simulink model "EDR100_Model4"  (R2023a)
settings: Solver=FixedStepAuto  StartTime=0  StopTime=t_end  FixedStep=h  RelTol=1e-3
InitFcn:
  | init_Model4
values from neighbouring files (symbols this model uses):
  A_f = 2.3    [init_Model4.m]
  c_d = 0.28    [init_Model4.m]
  c_r = 9.0/1000    (= 0.009)    [init_Model4.m]
  d_wheel = 2.101/pi*0.97    (= 0.648705998746)    [init_Model4.m]
  EM_inertia = 0    [init_Model4.m]
  EM_scaling = 1.8    [init_Model4.m]
  ESS_cell_Imax = ESS_cell_Cvalue*ESS_cell_Qmax    (= 15)    [init_Model4.m]
  ESS_cell_Imin = -ESS_cell_Cvalue*ESS_cell_Qmax    (= -15)    [init_Model4.m]
  ESS_cell_Qmax = 6    [init_Model4.m]
  ESS_cell_R10 = 0.4015*ESS_cell_R_scaling/ESS_cell_Emax    (= 0.0183333333333)    [init_Model4.m]
  ESS_cell_Vmax = 4.15    [init_Model4.m]
  ESS_cell_Vmin = 2.70    (= 2.7)    [init_Model4.m]
  ESS_cells_parallel = 58    [init_Model4.m]
  ESS_cells_series = 96    [init_Model4.m]
  ESS_pack_start_voltage = interp1(ESS_cell_OCV(2,:), ESS_cell_OCV(1,:),ESS_start_SOC ) * ESS_cells_series    [init_Model4.m]
  ESS_start_SOC = 80    [init_Model4.m]
  eta_gear = 0.98    [init_Model4.m]
  g = 9.81    [init_Model4.m]
  gear_ratio = 6    [init_Model4.m]
  h = 1.0    (= 1)    [init_Model4.m]
  m_v = 1832    [init_Model4.m]
  P_aux_EM = 0    [init_Model4.m]
  P_aux_gear = 0    [init_Model4.m]
  PEC_fs = 10000    [init_Model4.m]
  PEC_i2 = PEC_i2 * PEC_scaling    [init_Model4.m]
  PEC_Imax = PEC_Imax * PEC_scaling    [init_Model4.m]
  PEC_P_aux = 0    [init_Model4.m]
  PEC_phaseCount = 3    [init_Model4.m]
  PEC_Rd_con = PEC_Rd_con / PEC_scaling    [init_Model4.m]
  PEC_Rt_con = PEC_Rt_con / PEC_scaling    [init_Model4.m]
  PEC_Tj = 100    [init_Model4.m]
  PEC_U_DC = 400    [init_Model4.m]
  PEC_Umax = PEC_U_DC    (= 400)    [init_Model4.m]
  r_wheel = d_wheel/2    (= 0.324352999373)    [init_Model4.m]
  rho = 1.225    [init_Model4.m]
  rotating_mass = 0    [init_Model4.m]
  T_EM = linspace(y0,y1,ny)    [init_Model4.m]
  T_EM_max = T_EM_raw(:,1)    [init_Model4.m]
  w_EM = linspace(x0,x1,nx)'    [init_Model4.m]
  w_EM_max = w_EM_raw(:,end)    [init_Model4.m]
  w_EM_upper = max(max(w_EM_raw))    [init_Model4.m]
undefined symbols (not defined in the file or in its folder): ESS_cell_OCV, PEC_i1, PEC_Inom, PEC_J_ON_OFF_D, PEC_J_ON_OFF_T, PEC_scaling, PEC_T1, PEC_T2, PEC_v1, PEC_Vnom
Description:
  | Simulation model 4 (fourth lecture/assignment)
  | EDR100 "Electric Drive Systems", November 2022.
  | University West, Trollhättan, Sweden
  | Developed by Stefan Skoog
settings Model: Creator=Stefan  LastModifiedBy=victo
settings OptimizationCC: ReuseModelBlockBuffer=off
settings DebuggingCC: UnconnectedInputMsg=warning  UnconnectedOutputMsg=warning  UnconnectedLineMsg=warning
settings ModelReferenceCC: EnableRefExpFcnMdlSchedulingChecks=on
settings RTWCC: DLArmComputeVersion=19.05

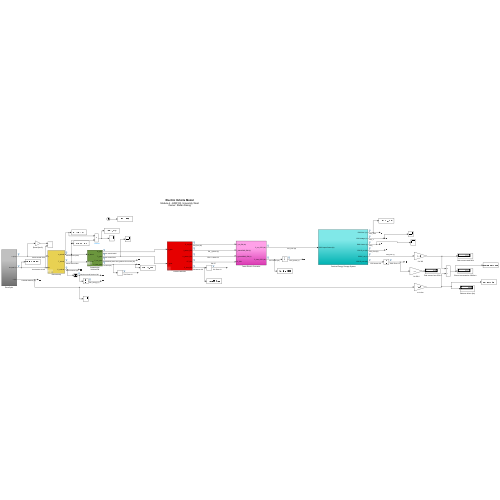
[thumbnail: Simulink's stored preview of the top-level diagram]
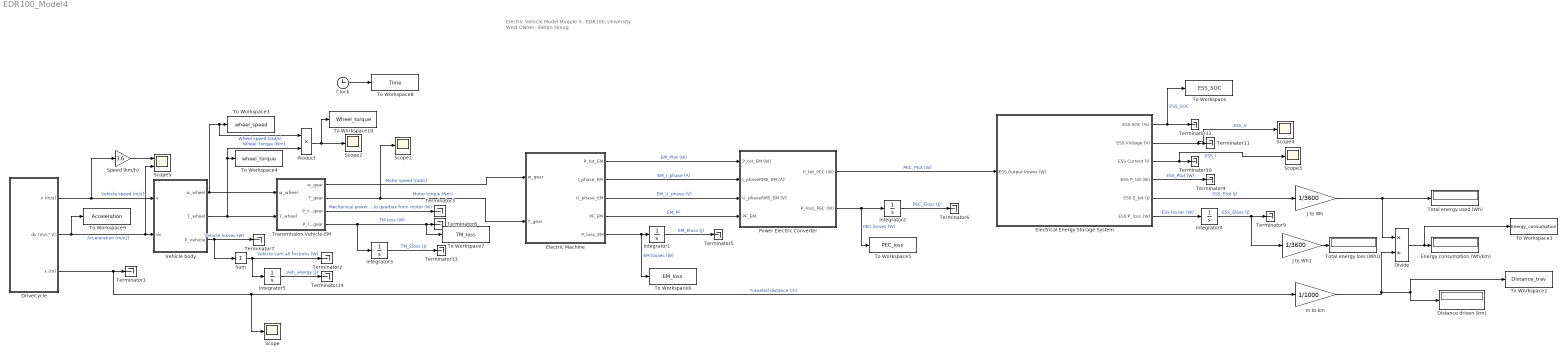
== system EDR100_Model4 ==
  note: Electric Vehicle Model
      | Module 4 - EDR100, University West
      | Owner: Stefan Skoog
  Clock : Clock
  Distance driven (km) : Display
  Divide : Product  Inputs=*/
  DriveCycle : Subsystem
  Electric Machine : Subsystem  mask{scale_EM=EM_scaling, theta_EM=EM_inertia, EM_P_aux=P_aux_EM}
      mask prompts: scale_EM "EM Scaling Factor (-)"; theta_EM "EM Inertia (kg*m²)"; EM_P_aux "Aux power (W)"
  Electrical Energy Storage System : Subsystem
  Energy consumption (Wh/km) : Display
  Integrator{1..5} (5 alike) : Integrator
  J to Wh : Gain  Gain=1/3600
  J to Wh1 : Gain  Gain=1/3600
  Power Electric Converter : Subsystem
  Product : Product  InputSameDT=on  RndMeth=Zero  SaturateOnIntegerOverflow=on  OutDataTypeStr=Inherit: Same as first input
  Scope{,1..4} (5 alike) : Scope
  Scope5 : Scope  NumInputPorts=2
  Speed (km/h) : Gain  Gain=3.6
  Sum : Sum  Inputs=+
  Terminator{1..14} (14 alike) : Terminator
  To Workspace : ToWorkspace  VariableName=ESS_SOC  SampleTime=-1
      settings: Save2DSignal=2-D array (concatenate along first dimension)
  To Workspace1 : ToWorkspace  VariableName=Energy_consumption  SampleTime=-1
      settings: Save2DSignal=2-D array (concatenate along first dimension)
  To Workspace10 : ToWorkspace  VariableName=Wheel_torque  SampleTime=-1
      settings: Save2DSignal=2-D array (concatenate along first dimension)
  To Workspace2 : ToWorkspace  VariableName=Distance_trav  SampleTime=-1
      settings: Save2DSignal=2-D array (concatenate along first dimension)
  To Workspace3 : ToWorkspace  VariableName=wheel_speed  SampleTime=-1
      settings: Save2DSignal=2-D array (concatenate along first dimension)
  To Workspace4 : ToWorkspace  VariableName=wheel_torque  SampleTime=-1
      settings: Save2DSignal=2-D array (concatenate along first dimension)
  To Workspace5 : ToWorkspace  VariableName=PEC_loss  SampleTime=-1
      settings: Save2DSignal=2-D array (concatenate along first dimension)
  To Workspace6 : ToWorkspace  VariableName=EM_loss  SampleTime=-1
      settings: Save2DSignal=2-D array (concatenate along first dimension)
  To Workspace7 : ToWorkspace  VariableName=TM_loss  SampleTime=-1
      settings: Save2DSignal=2-D array (concatenate along first dimension)
  To Workspace8 : ToWorkspace  VariableName=Time  SampleTime=-1
      settings: Save2DSignal=2-D array (concatenate along first dimension)
  To Workspace9 : ToWorkspace  VariableName=Acceleration  SampleTime=-1
      settings: Save2DSignal=2-D array (concatenate along first dimension)
  Total energy loss (Wh)1 : Display
  Total energy used (Wh) : Display
  Transmission Vehicle-EM : Subsystem  Tag=simple transmission  AncestorBlock=qss_tb_library/Gear System/Transmission  mask(Transmission){gear_ratio=gear_ratio, e_GT=eta_gear, P_GT0=P_aux_gear, w_wheel_min=1}
      mask prompts: gear_ratio "Gear ratio [-]"; e_GT "Efficiency [-]"; P_GT0 "Idling losses (friction) [W]"; w_wheel_min "Minimum wheel speed beyond which losses are generated [rad/s]"
      mask help:
      | This block simulates a transmission with a fixed gear ratio.
      |
      | Input:
      | =====
      | 	w_wheel	Speed of the wheel [rad/s]
      | 	dw_wheel	Acceleration of the wheel [rad/s^2]
      | 	T_wheel	Torque on the wheel [Nm]
      |
      | Output:
      | ======
      | 	w_trans		Speed of the fly wheel [rad/s]
      | 	dw_trans	Acceleration of the fly wheel [rad/s^2]
      | 	T_trans		Torque on the fly wheel [Nm]
  Vehicle body : Subsystem  Tag=vehicle  AncestorBlock=qss_tb_library/Vehicle/Vehicle  mask(Vehicle){m_f=m_v, mt2m_f=rotating_mass, A_f=A_f, d_wheel=d_wheel, cw=c_d, mu=c_r}
      mask prompts: m_f "Total mass of the vehicle [kg]"; mt2m_f "Rotating mass [%]"; A_f "Vehicle cross section [m^2]"; d_wheel "Wheel diameter [m]"; cw "Drag coefficient [-]"; mu "Rolling friction coefficient [-]"
      mask help:
      | This block computes the power required from the vehicle.
      |
      | Input:
      | =====
      | 	v		Speed [m/s]
      | 	dv		Acceleration [m/s^2]
      |
      | Output:
      | ======
      | 	w_wheel	Speed of the wheel [rad/s]
      | 	dw_wheel	Acceleration of the wheel [rad/s^2]
      | 	T_wheel	Torque on the wheel [Nm]
  m to km : Gain  Gain=1/1000
  wires:
  DriveCycle/2(dv (m/s^2)) -> Scope5/2, Vehicle body/2(dv), To Workspace9/1  "Acceleration (m/s2)"
  DriveCycle/1(v (m/s)) -> Vehicle body/1(v), Speed (km/h)/1  "Vehicle speed (m/s)"
  Vehicle body/1(w_wheel) -> Product/1, To Workspace3/1, Transmission Vehicle-EM/1(w_wheel)  "Wheel speed (rad/s)"
  Vehicle body/2(T_wheel) -> Product/2, To Workspace4/1, Transmission Vehicle-EM/2(T_wheel)  "Wheel Torque (Nm)"
  Vehicle body/3(P_vehicle) -> Terminator7/1, Sum/1  "Vehicle losses (W)"
  DriveCycle/3(x (m)) -> m to km/1, Scope/1, Terminator1/1  "Traveled distance (m)"
  Transmission Vehicle-EM/3(P_tot_gear) -> Terminator3/1  "Mechanical power into gearbox from motor (W)"
  Transmission Vehicle-EM/4(P_loss_gear) -> Integrator3/1, To Workspace7/1, Terminator8/1  "TM loss (W)"
  Integrator3/1 -> Terminator13/1  "TM_Eloss (J)"
  Transmission Vehicle-EM/2(T_gear) -> Scope1/1, Electric Machine/2(T_gear)  "Motor torque (Nm)"
  Integrator1/1 -> Terminator5/1  "EM_Eloss (J)"
  Electric Machine/5(P_loss_EM) -> To Workspace6/1, Integrator1/1  "EM losses (W)"
  Power Electric Converter/1(P_tot_PEC (W)) -> Electrical Energy Storage System/1(ESS Output Power (W))  "PEC_Ptot (W)"
  Electric Machine/1(P_tot_EM) -> Power Electric Converter/1(P_tot_EM (W))  "EM_Ptot (W)"
  Electric Machine/2(I_phase_EM) -> Power Electric Converter/2(I_phaseRMS_EM (A))  "EM_I_phase (A)"
  Electric Machine/3(U_phase_EM) -> Power Electric Converter/3(U_phaseRMS_EM (V))  "EM_U_phase (V)"
  Electric Machine/4(PF_EM) -> Power Electric Converter/4(PF_EM)  "EM_PF"
  Power Electric Converter/2(P_loss_PEC (W)) -> To Workspace5/1, Integrator2/1  "PEC losses (W)"
  Integrator2/1 -> Terminator6/1  "PEC_Eloss (J)"
  Integrator4/1 -> Terminator9/1, J to Wh1/1  "ESS_Eloss (J)"
  Electrical Energy Storage System/6(ESS P_loss (W)) -> Integrator4/1  "ESS losses (W)"
  Transmission Vehicle-EM/1(w_gear) -> Electric Machine/1(w_gear)  "Motor speed (rad/s)"
  m to km/1 -> Divide/2, Distance driven (km)/1, To Workspace2/1
  Electrical Energy Storage System/5(ESS E_tot (J)) -> J to Wh/1  "ESS_Etot (J)"
  J to Wh/1 -> Total energy used (Wh)/1, Divide/1
  Divide/1 -> To Workspace1/1, Energy consumption (Wh/km)/1
  Sum/1 -> Terminator2/1, Integrator5/1  "Vehicle sum all frictions (W)"
  Electrical Energy Storage System/4(ESS P_tot (W)) -> Terminator4/1  "ESS_Ptot (W)"
  Electrical Energy Storage System/2(ESS Voltage (V)) -> Scope4/1, Terminator11/1  "ESS_V"
  Electrical Energy Storage System/3(ESS Current (I)) -> Scope3/1, Terminator10/1  "ESS_I"
  Electrical Energy Storage System/1(ESS SOC (%)) -> To Workspace/1, Terminator12/1  "ESS_SOC"
  Integrator5/1 -> Terminator14/1  "Veh_energy (J)"
  Clock/1 -> To Workspace8/1
  J to Wh1/1 -> Total energy loss (Wh)1/1
  Product/1 -> To Workspace10/1, Scope2/1
  Speed (km/h)/1 -> Scope5/1

== system EDR100_Model4/DriveCycle ==
  Clock : Clock
  Differentiation : Subsystem
  Imported DriveCycle : FromWorkspace  VariableName=[t,v]  SampleTime=h  OutputAfterFinalValue=Setting to zero
  Integration : Subsystem
  To Workspace1 : ToWorkspace  VariableName=t  SampleTime=-1
  To Workspace2 : ToWorkspace  VariableName=x_tot  SampleTime=-1
  v (m/s) : Outport
  dv (m/s^2) : Outport  Port=2
  x (m) : Outport  Port=3  InitialOutput=0
  wires:
  Clock/1 -> To Workspace1/1  "Time (s)"
  Imported DriveCycle/1 -> Differentiation/1(V_z), Integration/1(V_z), v (m/s)/1  "Speed (m/s)"
  Integration/1(x_tot1) -> To Workspace2/1, x (m)/1  "Distance (m)"
  Differentiation/1(D_z) -> dv (m/s^2)/1  "Acceleration (m/s2)"

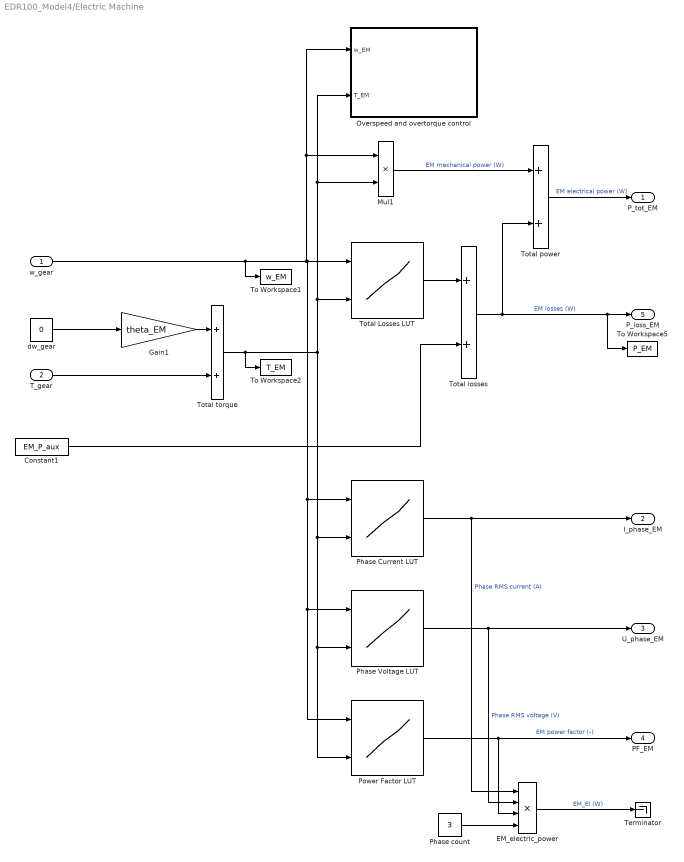
== system EDR100_Model4/Electric Machine ==
  w_gear : Inport
  T_gear : Inport  Port=2
  Constant1 : Constant  Value=EM_P_aux
  EM_electric_power : Product  Inputs=4
  Gain1 : Gain  Gain=theta_EM  SaturateOnIntegerOverflow=on  OutDataTypeStr=Inherit: Same as input  ParamDataTypeStr=Inherit: Same as input
  Mul1 : Product  Inputs=**
  Overspeed and overtorque control : Subsystem
  Phase Current LUT : Lookup_n-D  BreakpointsForDimension1=w_EM  BreakpointsForDimension2=T_EM  Table=Iph_EM_map'  ExtrapMethod=Clip  InternalRulePriority=Speed  RndMeth=Simplest
      settings: InputPortMap=u0,u1
  Phase Voltage LUT : Lookup_n-D  BreakpointsForDimension1=w_EM  BreakpointsForDimension2=T_EM  Table=Uph_EM_map'  ExtrapMethod=Clip  InternalRulePriority=Speed  RndMeth=Simplest
      settings: InputPortMap=u0,u1
  Phase count : Constant  Value=3
  Power Factor LUT : Lookup_n-D  BreakpointsForDimension1=w_EM  BreakpointsForDimension2=T_EM  Table=PF_EM_map'  ExtrapMethod=Clip  InternalRulePriority=Speed  RndMeth=Simplest
      settings: InputPortMap=u0,u1
  Terminator : Terminator
  To Workspace1 : ToWorkspace  VariableName=w_EM  SampleTime=-1
  To Workspace2 : ToWorkspace  VariableName=T_EM  SampleTime=-1
  To Workspace5 : ToWorkspace  VariableName=P_EM  SampleTime=-1
  Total Losses LUT : Lookup_n-D  BreakpointsForDimension1=w_EM  BreakpointsForDimension2=T_EM  Table=Loss_EM_map'  ExtrapMethod=Clip  InternalRulePriority=Speed  RndMeth=Simplest
      settings: InputPortMap=u0,u1
  Total losses : Sum  InputSameDT=on  SaturateOnIntegerOverflow=on  OutDataTypeStr=Inherit: Same as first input
  Total power : Sum  InputSameDT=on  SaturateOnIntegerOverflow=on  OutDataTypeStr=Inherit: Same as first input
  Total torque : Sum  InputSameDT=on  SaturateOnIntegerOverflow=on  OutDataTypeStr=Inherit: Same as first input
  dw_gear : Constant  Value=0
  P_tot_EM : Outport
  I_phase_EM : Outport  Port=2
  U_phase_EM : Outport  Port=3
  PF_EM : Outport  Port=4
  P_loss_EM : Outport  Port=5
  wires:
  T_gear/1 -> Total torque/2
  dw_gear/1 -> Gain1/1
  w_gear/1 -> To Workspace1/1, Total Losses LUT/1, Phase Current LUT/1, Power Factor LUT/1, Phase Voltage LUT/1, Overspeed and overtorque control/1(w_EM), Mul1/1
  Total losses/1 -> Total power/2, P_loss_EM/1, To Workspace5/1  "EM losses (W)"
  Total Losses LUT/1 -> Total losses/1
  Gain1/1 -> Total torque/1
  Total torque/1 -> Phase Current LUT/2, Power Factor LUT/2, Phase Voltage LUT/2, Total Losses LUT/2, Overspeed and overtorque control/2(T_EM), Mul1/2, To Workspace2/1
  Constant1/1 -> Total losses/2
  Phase Current LUT/1 -> I_phase_EM/1, EM_electric_power/1  "Phase RMS current (A)"
  Phase Voltage LUT/1 -> U_phase_EM/1, EM_electric_power/2  "Phase RMS voltage (V)"
  Total power/1 -> P_tot_EM/1  "EM electrical power (W)"
  Mul1/1 -> Total power/1  "EM mechanical power (W)"
  Power Factor LUT/1 -> PF_EM/1, EM_electric_power/3  "EM power factor (-)"
  EM_electric_power/1 -> Terminator/1  "EM_El (W)"
  Phase count/1 -> EM_electric_power/4

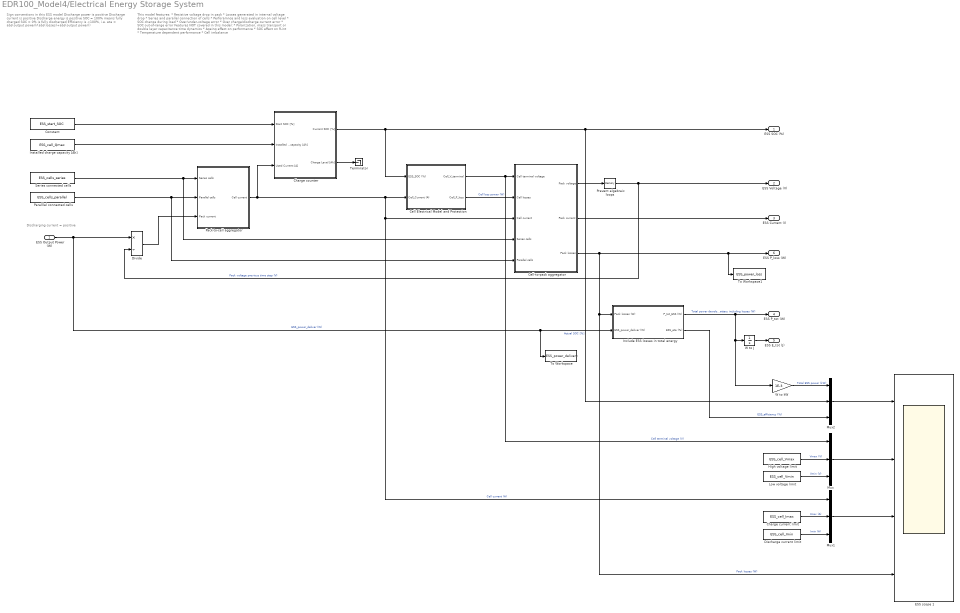
== system EDR100_Model4/Electrical Energy Storage System ==
  note: Discharging current = positive
  note: This model features:
      | * Resistive voltage drop in pack
      | * Losses generated in internal voltage drop
      | * Series and parallel connection of cells
      | * Perforamnce and loss evaluation on cell level
      | * SOC change during load
      | * Over/under-voltage error
      | * Over charge/discharge current error
      | * SOC out-of-range error
      |
      | Features NOT covered in this model:
      | * Polarization, mass transport or double layer capacitance time dynamics
      | * Ageing effect on performance
      | * SOC effect on R-int
      | * Temperature dependent performance
      | * Cell imbalance
  note: Sign conventions in this ESS model
      | Discharge power is positive
      | Discharge current is positive
      | Discharge energy is positive
      | SOC = 100% means fully charged
      | SOC = 0% is fully discharged
      | Efficiency is <100%, i.e.
      | eta = abs(output power)/(abs(losses)+abs(output power))
  ESS Output Power (W) : Inport
  Cell Electrical Model and Protection : Subsystem
  Cell-to-pack aggregator : Subsystem
  Charge counter : Subsystem
  Charge current limit : Constant  Value=ESS_cell_Imax
  Constant : Constant  Value=ESS_start_SOC
  Discharge current limit : Constant  Value=ESS_cell_Imin
  Divide : Product  Inputs=*/
  ESS scope 1 : Scope  NumInputPorts=4
  High voltage limit : Constant  Value=ESS_cell_Vmax
  Include ESS losses in total energy : Subsystem
  Installed charge capacity [Ah] : Constant  Value=ESS_cell_Qmax
  Low voltage limit : Constant  Value=ESS_cell_Vmin
  Mux : Mux  Inputs=3
  Mux1 : Mux  Inputs=3
  Mux2 : Mux  Inputs=3
  Pack-to-cell aggregator : Subsystem
  Paralllel connected cells : Constant  Value=ESS_cells_parallel
  Prevent algebraic loops : Memory  InitialCondition=ESS_pack_start_voltage
  Series connected cells : Constant  Value=ESS_cells_series
  Terminator : Terminator
  To Workspace : ToWorkspace  VariableName=ESS_power_delivery  SampleTime=-1
      settings: Save2DSignal=2-D array (concatenate along first dimension)
  To Workspace1 : ToWorkspace  VariableName=ESS_power_loss  SampleTime=-1
      settings: Save2DSignal=2-D array (concatenate along first dimension)
  W to J : Integrator
  W to kW : Gain  Gain=1E-3
  ESS SOC (%) : Outport
  ESS Voltage (V) : Outport  Port=2
  ESS Current (I) : Outport  Port=3
  ESS P_tot (W) : Outport  Port=4
  ESS E_tot (J) : Outport  Port=5
  ESS P_loss (W) : Outport  Port=6
  wires:
  Series connected cells/1 -> Cell-to-pack aggregator/4(Series cells), Pack-to-cell aggregator/1(Series cells)
  Pack-to-cell aggregator/1(Cell current) -> Mux1/1, Cell-to-pack aggregator/3(Cell current), Cell Electrical Model and Protection/2(Cell_Current (A)), Charge counter/3(Used Current [A])  "Cell current (A)"
  Installed charge capacity [Ah]/1 -> Charge counter/2(Installed charge capacity [Ah])
  Constant/1 -> Charge counter/1(Start SOC [%])
  Divide/1 -> Pack-to-cell aggregator/3(Pack current)
  Paralllel connected cells/1 -> Cell-to-pack aggregator/5(Parallel cells), Pack-to-cell aggregator/2(Parallel cells)
  Charge counter/1(Current SOC [%]) -> ESS SOC (%)/1, Mux2/2, Cell Electrical Model and Protection/1(ESS_SOC (%))  "Actual SOC [%]"
  Charge counter/2(Charge Level [Ah]) -> Terminator/1
  Cell Electrical Model and Protection/1(Cell_V_terminal) -> Mux/1, Cell-to-pack aggregator/1(Cell terminal voltage)  "Cell terminal voltage (V)"
  Cell Electrical Model and Protection/2(Cell_P_loss) -> Cell-to-pack aggregator/2(Cell losses)  "Cell loss power (W)"
  Cell-to-pack aggregator/3(Pack losses) -> To Workspace1/1, ESS P_loss (W)/1, Include ESS losses in total energy/1(Pack losses (W)), ESS scope 1/4  "Pack losses (W)"
  Cell-to-pack aggregator/1(Pack voltage) -> Prevent algebraic loops/1
  Prevent algebraic loops/1 -> ESS Voltage (V)/1, Divide/2  "Pack voltage previous time step (V)"
  Cell-to-pack aggregator/2(Pack current) -> ESS Current (I)/1
  ESS Output Power (W)/1 -> Divide/1, To Workspace/1, Include ESS losses in total energy/2(ESS_power_deliver (W))  "ESS_power_deliver (W)"
  Mux2/1 -> ESS scope 1/1
  Mux/1 -> ESS scope 1/2
  Mux1/1 -> ESS scope 1/3
  W to J/1 -> ESS E_tot (J)/1
  Include ESS losses in total energy/1(P_tot_ESS (W)) -> ESS P_tot (W)/1, W to kW/1, W to J/1  "Total power developed in battery including losses (W)"
  Charge current limit/1 -> Mux1/2  "Imax (A)"
  High voltage limit/1 -> Mux/2  "Vmax (V)"
  Discharge current limit/1 -> Mux1/3  "Imin (A)"
  Low voltage limit/1 -> Mux/3  "Vmin (V)"
  Include ESS losses in total energy/2(ESS_eta (%)) -> Mux2/3  "ESS_efficiency (%)"
  W to kW/1 -> Mux2/1  "Total ESS power (kW)"

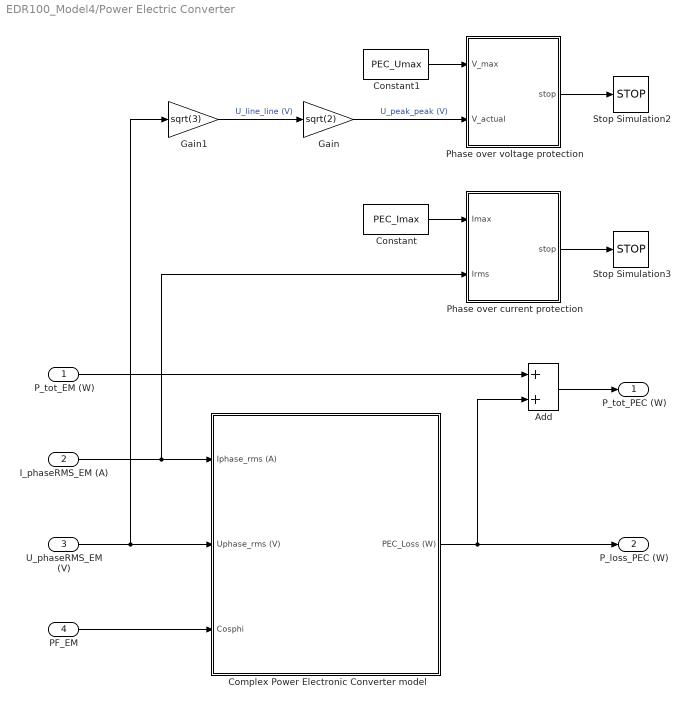
== system EDR100_Model4/Power Electric Converter ==
  P_tot_EM (W) : Inport
  I_phaseRMS_EM (A) : Inport  Port=2
  U_phaseRMS_EM (V) : Inport  Port=3
  PF_EM : Inport  Port=4
  Add : Sum
  Complex Power Electronic Converter model : Subsystem  mask(3-phase IGBT inverter){scale_PEC=PEC_scaling, Udc=PEC_U_DC, fsw=PEC_fs, Tjunct=PEC_Tj, LV_Losses=PEC_P_aux}
      mask prompts: scale_PEC "PEC Scaling Factor (-)"; Udc "Supply direct voltage level (V)"; fsw "Switching frequency (Hz)"; Tjunct "IGBT Junction temperature (°C)"; LV_Losses "Aux losses (W)"
      mask help:
      | This blocks simulates losses for a three-leg, two-level converter based on forward conduction losses and diod losses in IGBT modules.
      |
      | Input:
      | =====
      | I_phaseRMS		Phase RMS current of electric machine (V)
      | U_phaseRMS		Phase RMS voltage of electric machine (V)
      | cosphi			Power factor [0..1] of electric machine (-)
      |
      | Ouput:
      | ======
      | Pinv	Total losses in inverter (W)
  Constant : Constant  Value=PEC_Imax
  Constant1 : Constant  Value=PEC_Umax
  Gain : Gain  Gain=sqrt(2)
  Gain1 : Gain  Gain=sqrt(3)
  Phase over current protection : MATLAB Function  TreatAsAtomicUnit=on
  Phase over voltage protection : MATLAB Function  TreatAsAtomicUnit=on
  Stop Simulation2 : Stop
  Stop Simulation3 : Stop
  P_tot_PEC (W) : Outport
  P_loss_PEC (W) : Outport  Port=2
  wires:
  Constant/1 -> Phase over current protection/1(Imax)
  Constant1/1 -> Phase over voltage protection/1(V_max)
  PF_EM/1 -> Complex Power Electronic Converter model/3(Cosphi)
  P_tot_EM (W)/1 -> Add/1
  Phase over current protection/1(stop) -> Stop Simulation3/1
  Add/1 -> P_tot_PEC (W)/1
  Gain1/1 -> Gain/1  "U_line_line (V)"
  Phase over voltage protection/1(stop) -> Stop Simulation2/1
  Gain/1 -> Phase over voltage protection/2(V_actual)  "U_peak_peak (V)"
  U_phaseRMS_EM (V)/1 -> Gain1/1, Complex Power Electronic Converter model/2(Uphase_rms (V))
  I_phaseRMS_EM (A)/1 -> Phase over current protection/2(Irms), Complex Power Electronic Converter model/1(Iphase_rms (A))
  Complex Power Electronic Converter model/1(PEC_Loss (W)) -> Add/2, P_loss_PEC (W)/1

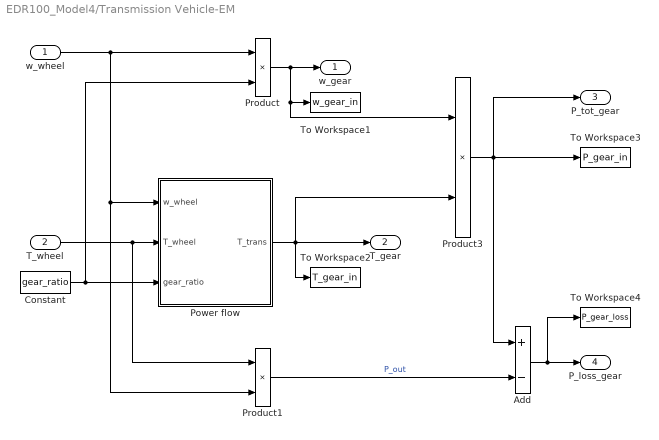
== system EDR100_Model4/Transmission Vehicle-EM ==
  w_wheel : Inport
  T_wheel : Inport  Port=2
  Add : Sum  Inputs=+-
  Constant : Constant  Value=gear_ratio
  Power flow : Subsystem
  Product : Product  InputSameDT=on  RndMeth=Zero  SaturateOnIntegerOverflow=on  OutDataTypeStr=Inherit: Same as first input
  Product1 : Product  InputSameDT=on  RndMeth=Zero  SaturateOnIntegerOverflow=on  OutDataTypeStr=Inherit: Same as first input
  Product3 : Product  InputSameDT=on  RndMeth=Zero  SaturateOnIntegerOverflow=on  OutDataTypeStr=Inherit: Same as first input
  To Workspace1 : ToWorkspace  VariableName=w_gear_in  SampleTime=-1
  To Workspace2 : ToWorkspace  VariableName=T_gear_in  SampleTime=-1
  To Workspace3 : ToWorkspace  VariableName=P_gear_in  SampleTime=-1
  To Workspace4 : ToWorkspace  VariableName=P_gear_loss  SampleTime=-1
  w_gear : Outport  InitialOutput=0
  T_gear : Outport  Port=2  InitialOutput=0
  P_tot_gear : Outport  Port=3  InitialOutput=0
  P_loss_gear : Outport  Port=4  InitialOutput=0
  wires:
  Product3/1 -> P_tot_gear/1, To Workspace3/1, Add/1
  w_wheel/1 -> Product1/2, Power flow/1(w_wheel), Product/1
  Constant/1 -> Product/2, Power flow/3(gear_ratio)
  T_wheel/1 -> Product1/1, Power flow/2(T_wheel)
  Product/1 -> Product3/1, To Workspace1/1, w_gear/1
  Power flow/1(T_trans) -> Product3/2, To Workspace2/1, T_gear/1
  Product1/1 -> Add/2  "P_out"
  Add/1 -> To Workspace4/1, P_loss_gear/1

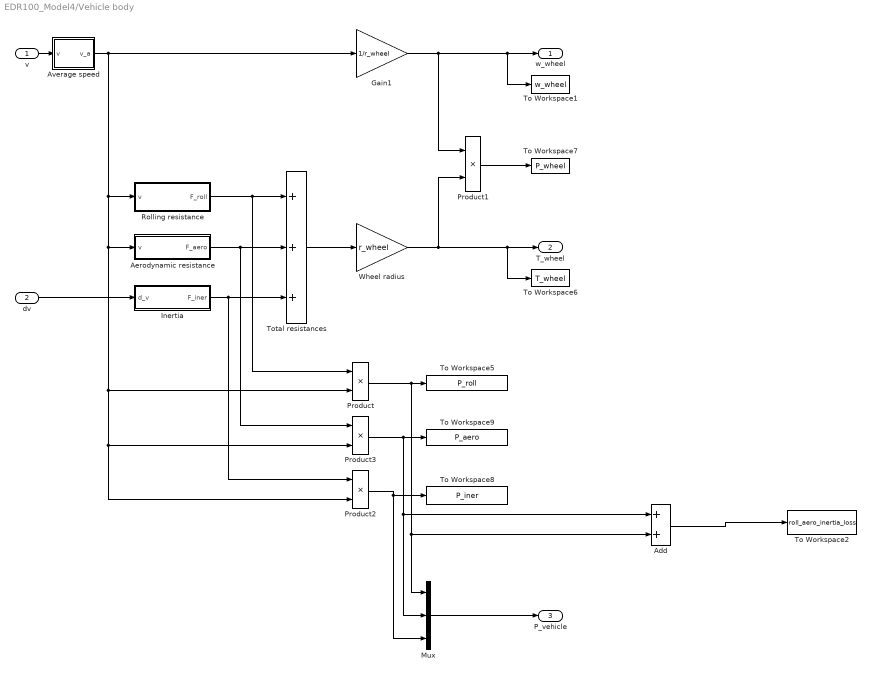
== system EDR100_Model4/Vehicle body ==
  v : Inport
  dv : Inport  Port=2
  Add : Sum
  Aerodynamic resistance : Subsystem
  Average speed : Subsystem
  Gain1 : Gain  Gain=1/r_wheel  SaturateOnIntegerOverflow=on  OutDataTypeStr=Inherit: Same as input  ParamDataTypeStr=Inherit: Same as input
  Inertia : Subsystem
  Mux : Mux  Inputs=3
  Product{,1..3} (4 alike) : Product  InputSameDT=on  RndMeth=Zero  SaturateOnIntegerOverflow=on  OutDataTypeStr=Inherit: Same as first input
  Rolling resistance : Subsystem
  To Workspace1 : ToWorkspace  VariableName=w_wheel  SampleTime=-1
  To Workspace2 : ToWorkspace  VariableName=roll_aero_inertia_loss  SampleTime=-1
      settings: Save2DSignal=2-D array (concatenate along first dimension)
  To Workspace5 : ToWorkspace  VariableName=P_roll  SampleTime=-1
  To Workspace6 : ToWorkspace  VariableName=T_wheel  SampleTime=-1
  To Workspace7 : ToWorkspace  VariableName=P_wheel  SampleTime=-1
  To Workspace8 : ToWorkspace  VariableName=P_iner  SampleTime=-1
  To Workspace9 : ToWorkspace  VariableName=P_aero  SampleTime=-1
  Total resistances : Sum  Inputs=+++  InputSameDT=on  SaturateOnIntegerOverflow=on  OutDataTypeStr=Inherit: Same as first input
  Wheel radius : Gain  Gain=r_wheel  SaturateOnIntegerOverflow=on  OutDataTypeStr=Inherit: Same as input  ParamDataTypeStr=Inherit: Same as input
  w_wheel : Outport  InitialOutput=0
  T_wheel : Outport  Port=2  InitialOutput=0
  P_vehicle : Outport  Port=3  InitialOutput=0
  wires:
  Product/1 -> To Workspace5/1, Add/2, Mux/1
  Product1/1 -> To Workspace7/1
  Product3/1 -> Mux/2, Add/1, To Workspace9/1
  Product2/1 -> Mux/3, To Workspace8/1
  v/1 -> Average speed/1(v)
  dv/1 -> Inertia/1(d_v)
  Wheel radius/1 -> Product1/2, To Workspace6/1, T_wheel/1
  Total resistances/1 -> Wheel radius/1
  Inertia/1(F_iner) -> Product2/1, Total resistances/3
  Aerodynamic resistance/1(F_aero) -> Total resistances/2, Product3/1
  Rolling resistance/1(F_roll) -> Product/1, Total resistances/1
  Gain1/1 -> To Workspace1/1, w_wheel/1, Product1/1
  Average speed/1(v_a) -> Product/2, Product2/2, Product3/2, Aerodynamic resistance/1(v), Rolling resistance/1(v), Gain1/1
  Mux/1 -> P_vehicle/1
  Add/1 -> To Workspace2/1

== system EDR100_Model4/DriveCycle/Differentiation ==
  V_z : Inport
  Sum1 : Sum  Inputs=+-  InputSameDT=on  SaturateOnIntegerOverflow=on  OutDataTypeStr=Inherit: Same as first input
  Unit Delay1 : UnitDelay  SampleTime=h
  D_z : Outport  InitialOutput=0
  wires:
  Unit Delay1/1 -> Sum1/2
  V_z/1 -> Sum1/1, Unit Delay1/1
  Sum1/1 -> D_z/1

== system EDR100_Model4/DriveCycle/Integration ==
  V_z : Inport
  Gain4 : Gain  Gain=0.5*h  SaturateOnIntegerOverflow=on  OutDataTypeStr=Inherit: Same as input  ParamDataTypeStr=Inherit: Same as input
  Plant : UnitDelay  InitialCondition=1  SampleTime=h
  Sum2 : Sum  InputSameDT=on  SaturateOnIntegerOverflow=on  OutDataTypeStr=Inherit: Same as first input
  Sum4 : Sum  InputSameDT=on  SaturateOnIntegerOverflow=on  OutDataTypeStr=Inherit: Same as first input
  Unit Delay2 : UnitDelay  SampleTime=h
  x_tot1 : Outport  InitialOutput=0
  wires:
  Unit Delay2/1 -> Sum2/2
  Sum2/1 -> Gain4/1
  Gain4/1 -> Sum4/2
  Plant/1 -> x_tot1/1, Sum4/1
  V_z/1 -> Sum2/1, Unit Delay2/1
  Sum4/1 -> Plant/1

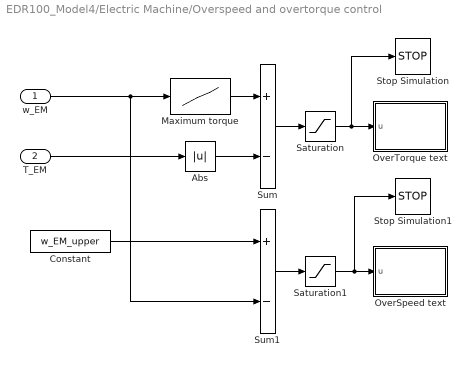
== system EDR100_Model4/Electric Machine/Overspeed and overtorque control ==
  w_EM : Inport
  T_EM : Inport  Port=2
  Abs : Abs
  Constant : Constant  Value=w_EM_upper
  Maximum torque : Lookup  InputValues=w_EM_max  Table=T_EM_max
  OverSpeed text : MATLAB Function  TreatAsAtomicUnit=on
  OverTorque text : MATLAB Function  TreatAsAtomicUnit=on
  Saturation : Saturate  UpperLimit=0  LowerLimit=-inf
  Saturation1 : Saturate  UpperLimit=0  LowerLimit=-inf
  Stop Simulation : Stop
  Stop Simulation1 : Stop
  Sum : Sum  Inputs=+-  InputSameDT=on  SaturateOnIntegerOverflow=on  OutDataTypeStr=Inherit: Same as first input
  Sum1 : Sum  Inputs=+-  InputSameDT=on  SaturateOnIntegerOverflow=on  OutDataTypeStr=Inherit: Same as first input
  wires:
  Saturation/1 -> Stop Simulation/1, OverTorque text/1(u)
  Constant/1 -> Sum1/1
  w_EM/1 -> Maximum torque/1, Sum1/2
  Abs/1 -> Sum/2
  Saturation1/1 -> Stop Simulation1/1, OverSpeed text/1(u)
  Sum1/1 -> Saturation1/1
  T_EM/1 -> Abs/1
  Maximum torque/1 -> Sum/1
  Sum/1 -> Saturation/1

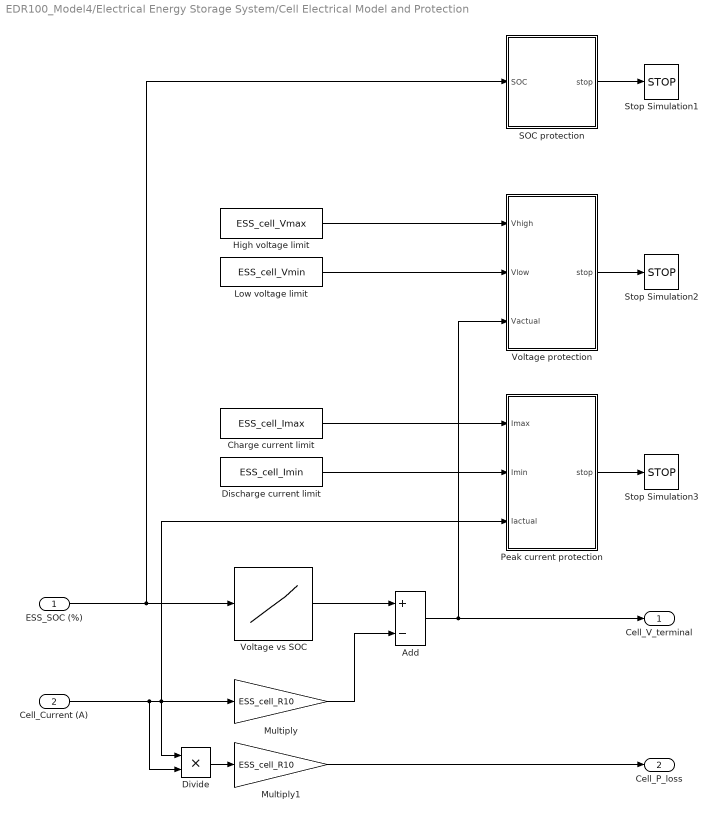
== system EDR100_Model4/Electrical Energy Storage System/Cell Electrical Model and Protection ==
  ESS_SOC (%) : Inport
  Cell_Current (A) : Inport  Port=2
  Add : Sum  Inputs=+-
  Charge current limit : Constant  Value=ESS_cell_Imax
  Discharge current limit : Constant  Value=ESS_cell_Imin
  Divide : Product  Inputs=**
  High voltage limit : Constant  Value=ESS_cell_Vmax
  Low voltage limit : Constant  Value=ESS_cell_Vmin
  Multiply : Gain  Gain=ESS_cell_R10
  Multiply1 : Gain  Gain=ESS_cell_R10
  Peak current protection : MATLAB Function  TreatAsAtomicUnit=on
  SOC protection : MATLAB Function  TreatAsAtomicUnit=on
  Stop Simulation1 : Stop
  Stop Simulation2 : Stop
  Stop Simulation3 : Stop
  Voltage protection : MATLAB Function  TreatAsAtomicUnit=on
  Voltage vs SOC : Lookup_n-D  NumberOfTableDimensions=1  BreakpointsForDimension1=ESS_cell_OCV(2,:)  Table=ESS_cell_OCV(1,:)  InternalRulePriority=Speed  RndMeth=Simplest
  Cell_V_terminal : Outport
  Cell_P_loss : Outport  Port=2
  wires:
  ESS_SOC (%)/1 -> SOC protection/1(SOC), Voltage vs SOC/1
  Cell_Current (A)/1 -> Divide/2, Divide/1, Multiply/1, Peak current protection/3(Iactual)
  Voltage vs SOC/1 -> Add/1
  Multiply/1 -> Add/2
  Add/1 -> Voltage protection/3(Vactual), Cell_V_terminal/1
  Multiply1/1 -> Cell_P_loss/1
  Divide/1 -> Multiply1/1
  Voltage protection/1(stop) -> Stop Simulation2/1
  Low voltage limit/1 -> Voltage protection/2(Vlow)
  High voltage limit/1 -> Voltage protection/1(Vhigh)
  SOC protection/1(stop) -> Stop Simulation1/1
  Charge current limit/1 -> Peak current protection/1(Imax)
  Discharge current limit/1 -> Peak current protection/2(Imin)
  Peak current protection/1(stop) -> Stop Simulation3/1

== system EDR100_Model4/Electrical Energy Storage System/Cell-to-pack aggregator ==
  Cell terminal voltage : Inport
  Cell losses : Inport  Port=2
  Cell current : Inport  Port=3
  Series cells : Inport  Port=4
  Parallel cells : Inport  Port=5
  Mul1 : Product  Inputs=**
  Mul2 : Product  Inputs=**
  Mul3 : Product  Inputs=***
  Pack voltage : Outport
  Pack current : Outport  Port=2
  Pack losses : Outport  Port=3
  wires:
  Mul1/1 -> Pack voltage/1
  Mul2/1 -> Pack current/1
  Cell terminal voltage/1 -> Mul1/1
  Cell current/1 -> Mul2/1
  Parallel cells/1 -> Mul2/2, Mul3/2
  Series cells/1 -> Mul3/1, Mul1/2
  Mul3/1 -> Pack losses/1
  Cell losses/1 -> Mul3/3

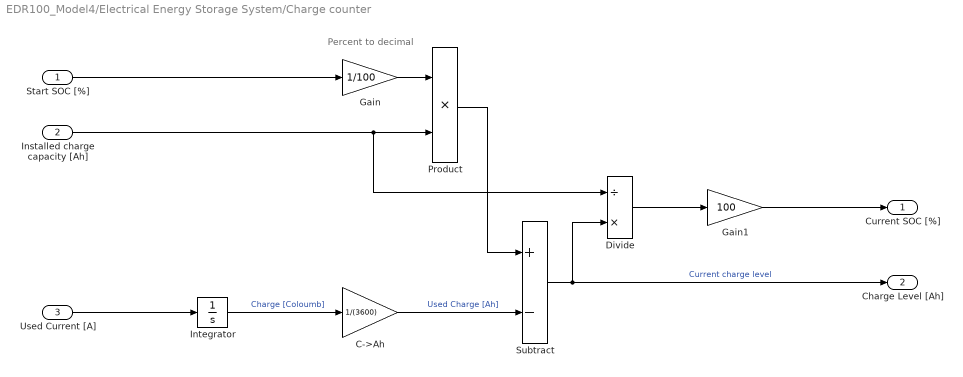
== system EDR100_Model4/Electrical Energy Storage System/Charge counter ==
  note: Percent to decimal
  Start SOC [%] : Inport
  Installed charge capacity [Ah] : Inport  Port=2
  Used Current [A] : Inport  Port=3
  C->Ah : Gain  Gain=1/(3600)
  Divide : Product  Inputs=/*
  Gain : Gain  Gain=1/100
  Gain1 : Gain  Gain=100
  Integrator : Integrator
  Product : Product
  Subtract : Sum  Inputs=+-
  Current SOC [%] : Outport
  Charge Level [Ah] : Outport  Port=2
  wires:
  Subtract/1 -> Divide/2, Charge Level [Ah]/1  "Current charge level"
  Integrator/1 -> C->Ah/1  "Charge [Coloumb]"
  C->Ah/1 -> Subtract/2  "Used Charge [Ah]"
  Gain/1 -> Product/1
  Installed charge capacity [Ah]/1 -> Divide/1, Product/2
  Start SOC [%]/1 -> Gain/1
  Used Current [A]/1 -> Integrator/1
  Product/1 -> Subtract/1
  Divide/1 -> Gain1/1
  Gain1/1 -> Current SOC [%]/1

== system EDR100_Model4/Electrical Energy Storage System/Include ESS losses in total energy ==
  Pack losses (W) : Inport
  ESS_power_deliver (W) : Inport  Port=2
  Add losses to total internal power : Sum
  Divide1 : Product  Inputs=/*
  Mul : Product  Inputs=**
  Polarity of delivered power : Signum
  to Percent : Gain  Gain=100
  P_tot_ESS (W) : Outport
  ESS_eta (%) : Outport  Port=2
  wires:
  Polarity of delivered power/1 -> Mul/2
  ESS_power_deliver (W)/1 -> Divide1/2, Polarity of delivered power/1, Add losses to total internal power/2
  Mul/1 -> Add losses to total internal power/1
  Add losses to total internal power/1 -> Divide1/1, P_tot_ESS (W)/1  "P_tot_ESS (W)"
  Pack losses (W)/1 -> Mul/1
  Divide1/1 -> to Percent/1
  to Percent/1 -> ESS_eta (%)/1  "ESS efficiency (%)"

== system EDR100_Model4/Electrical Energy Storage System/Pack-to-cell aggregator ==
  Series cells : Inport
  Parallel cells : Inport  Port=2
  Pack current : Inport  Port=3
  Divide2 : Product  Inputs=*/
  Terminator3 : Terminator
  Cell current : Outport
  wires:
  Pack current/1 -> Divide2/1
  Parallel cells/1 -> Divide2/2
  Divide2/1 -> Cell current/1
  Series cells/1 -> Terminator3/1

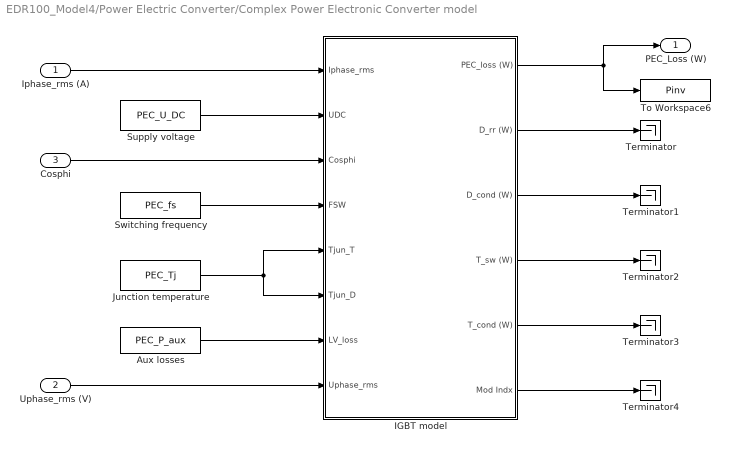
== system EDR100_Model4/Power Electric Converter/Complex Power Electronic Converter model ==
  Iphase_rms (A) : Inport
  Uphase_rms (V) : Inport  Port=2
  Cosphi : Inport  Port=3
  Aux losses : Constant  Value=PEC_P_aux
  IGBT model : Subsystem
  Junction temperature : Constant  Value=PEC_Tj
  Supply voltage : Constant  Value=PEC_U_DC
  Switching frequency : Constant  Value=PEC_fs
  Terminator{,1..4} (5 alike) : Terminator
  To Workspace6 : ToWorkspace  VariableName=Pinv  SampleTime=-1
  PEC_Loss (W) : Outport
  wires:
  IGBT model/1(PEC_loss (W)) -> To Workspace6/1, PEC_Loss (W)/1
  IGBT model/3("D_cond (W) ") -> Terminator1/1
  Junction temperature/1 -> IGBT model/6(Tjun_D), IGBT model/5(Tjun_T)
  Switching frequency/1 -> IGBT model/4(FSW)
  Supply voltage/1 -> IGBT model/2(UDC)
  Cosphi/1 -> IGBT model/3(Cosphi)
  Aux losses/1 -> IGBT model/7("LV_loss ")
  IGBT model/2("D_rr (W) ") -> Terminator/1
  IGBT model/6(Mod Indx) -> Terminator4/1
  IGBT model/4(T_sw (W)) -> Terminator2/1
  IGBT model/5(T_cond (W)) -> Terminator3/1
  Iphase_rms (A)/1 -> IGBT model/1(Iphase_rms)
  Uphase_rms (V)/1 -> IGBT model/8(Uphase_rms)

== system EDR100_Model4/Transmission Vehicle-EM/Power flow ==
  w_wheel : Inport
  T_wheel : Inport  Port=2
  gear_ratio : Inport  Port=3
  "Energy Engine -> Wheel" : Subsystem
  "Energy Wheel -> Engine" : Subsystem
  Switch1 : Switch
  T_trans : Outport  InitialOutput=0
  wires:
  Switch1/1 -> T_trans/1
  "Energy Engine -> Wheel"/1(T_trans+) -> Switch1/1
  T_wheel/1 -> Switch1/2, "Energy Engine -> Wheel"/2(T_wheel), "Energy Wheel -> Engine"/2(T_wheel)
  "Energy Wheel -> Engine"/1(T_trans-) -> Switch1/3
  gear_ratio/1 -> "Energy Engine -> Wheel"/3(gear_ratio), "Energy Wheel -> Engine"/3(gear_ratio)
  w_wheel/1 -> "Energy Engine -> Wheel"/1(w_wheel), "Energy Wheel -> Engine"/1(w_wheel)

== system EDR100_Model4/Vehicle body/Aerodynamic resistance ==
  v : Inport
  Aerodynamic resistance : Fcn  Expr=0.5*rho*cw*A_f*u^2
  To Workspace10 : ToWorkspace  VariableName=F_aero  SampleTime=-1
  F_aero : Outport  InitialOutput=0
  wires:
  Aerodynamic resistance/1 -> To Workspace10/1, F_aero/1
  v/1 -> Aerodynamic resistance/1

== system EDR100_Model4/Vehicle body/Average speed ==
  v : Inport
  Gain5 : Gain  Gain=0.5  SaturateOnIntegerOverflow=on  OutDataTypeStr=Inherit: Same as input  ParamDataTypeStr=Inherit: Same as input
  Sum2 : Sum  InputSameDT=on  SaturateOnIntegerOverflow=on  OutDataTypeStr=Inherit: Same as first input
  Unit Delay : UnitDelay  SampleTime=h
  v_a : Outport  InitialOutput=0
  wires:
  v/1 -> Unit Delay/1, Sum2/1
  Gain5/1 -> v_a/1
  Sum2/1 -> Gain5/1
  Unit Delay/1 -> Sum2/2

== system EDR100_Model4/Vehicle body/Inertia ==
  d_v : Inport
  Inertia : Fcn  Expr=m_f*(1+mt2m_f)*u/h
  To Workspace10 : ToWorkspace  VariableName=F_iner  SampleTime=-1
  F_iner : Outport  InitialOutput=0
  wires:
  d_v/1 -> Inertia/1
  Inertia/1 -> To Workspace10/1, F_iner/1

== system EDR100_Model4/Vehicle body/Rolling resistance ==
  v : Inport
  Constant : Constant  Value=m_f
  Constant1 : Constant  Value=g
  Constant2 : Constant  Value=c_r
  Divide : Product  Inputs=***
  Switch : Switch  Criteria=u2 > Threshold  Threshold=eps  SaturateOnIntegerOverflow=off  InputSameDT=off
  To Workspace2 : ToWorkspace  VariableName=F_roll  SampleTime=-1
  standstill : Constant  Value=0
  F_roll : Outport
  wires:
  standstill/1 -> Switch/3
  v/1 -> Switch/2
  Switch/1 -> F_roll/1, To Workspace2/1
  Constant/1 -> Divide/1
  Constant1/1 -> Divide/2
  Constant2/1 -> Divide/3
  Divide/1 -> Switch/1

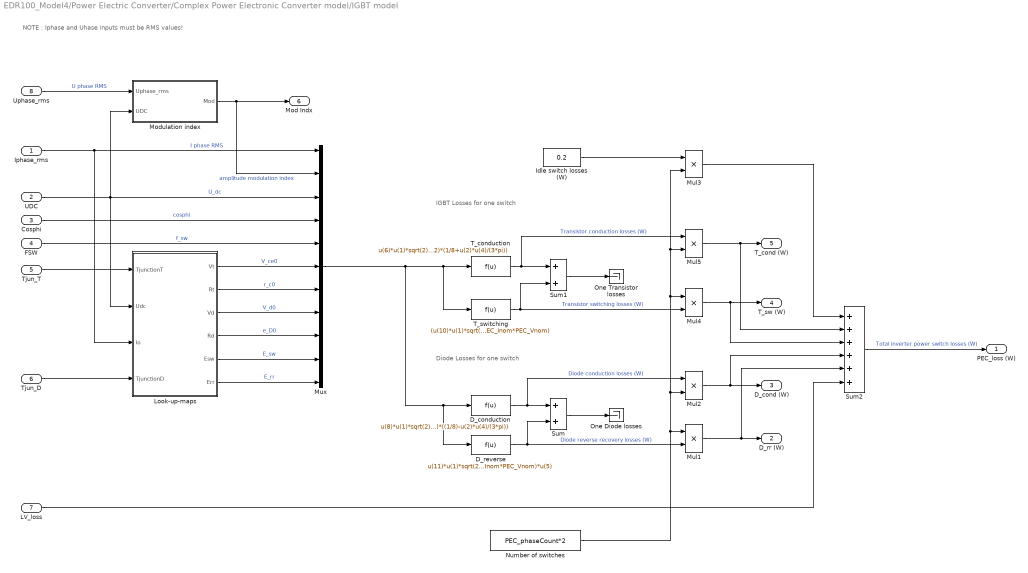
== system EDR100_Model4/Power Electric Converter/Complex Power Electronic Converter model/IGBT model ==
  note: NOTE :
      | Iphase and Uhase inputs must be RMS values!
  note: IGBT Losses for one switch
  note: Diode Losses for one switch
  Iphase_rms : Inport
  UDC : Inport  Port=2
  Cosphi : Inport  Port=3
  FSW : Inport  Port=4
  Tjun_T : Inport  Port=5
  Tjun_D : Inport  Port=6
  "LV_loss " : Inport  Port=7
  Uphase_rms : Inport  Port=8
  D_conduction : Fcn  Expr=u(8)*u(1)*sqrt(2)*(1/(2*pi)-u(2)*u(4)/8)+u(9)*(u(1)*sqrt(2)^2)*((1/8)-u(2)*u(4)/(3*pi))
  D_reverse : Fcn  Expr=u(11)*u(1)*sqrt(2)*u(3)/(pi*PEC_Inom*PEC_Vnom)*u(5)
  Idle switch losses (W) : Constant  Value=0.2
  Look-up-maps : Subsystem
  "Modulation index " : Subsystem
  Mul{1..5} (5 alike) : Product  Inputs=**
  Mux : Mux  Inputs=11
  Number of switches : Constant  Value=PEC_phaseCount*2
  One Diode losses : Terminator
  One Transistor losses : Terminator
  Sum : Sum
  Sum1 : Sum
  Sum2 : Sum  Inputs=++++++
  T_conduction : Fcn  Expr=u(6)*u(1)*sqrt(2)*(1/(2*pi)+u(2)*u(4)/8)+u(7)*(u(1)*sqrt(2)^2)*(1/8+u(2)*u(4)/(3*pi))
  T_switching : Fcn  Expr=(u(10)*u(1)*sqrt(2)*u(3)*u(5))/(pi*PEC_Inom*PEC_Vnom)
  PEC_loss (W) : Outport
  "D_rr (W) " : Outport  Port=2
  "D_cond (W) " : Outport  Port=3
  T_sw (W) : Outport  Port=4
  T_cond (W) : Outport  Port=5
  Mod Indx : Outport  Port=6
  wires:
  Mul1/1 -> Sum2/5, "D_rr (W) "/1
  Tjun_T/1 -> Look-up-maps/1(TjunctionT)
  Look-up-maps/5(Esw) -> Mux/10  "E_sw"
  Mul2/1 -> Sum2/4, "D_cond (W) "/1
  Cosphi/1 -> Mux/4  "cosphi"
  FSW/1 -> Mux/5  "f_sw"
  Look-up-maps/4(Rd) -> Mux/9  "e_D0"
  Iphase_rms/1 -> Mux/1, Look-up-maps/3("Io ")  "I phase RMS"
  D_reverse/1 -> Sum/2, Mul1/2  "Diode reverse recovery losses (W)"
  T_switching/1 -> Sum1/2, Mul4/2  "Transistor switching losses (W)"
  Look-up-maps/2(Rt) -> Mux/7  "r_c0"
  "Modulation index "/1(Mod) -> Mux/2, Mod Indx/1  "amplitude modulation index"
  "LV_loss "/1 -> Sum2/6
  Look-up-maps/1(Vt) -> Mux/6  "V_ce0"
  D_conduction/1 -> Mul2/1, Sum/1  "Diode conduction losses (W)"
  Look-up-maps/6(Err) -> Mux/11  "E_rr"
  Mul4/1 -> Sum2/3, T_sw (W)/1
  Mul5/1 -> Sum2/2, T_cond (W)/1
  Mux/1 -> D_reverse/1, D_conduction/1, T_switching/1, T_conduction/1
  Tjun_D/1 -> Look-up-maps/4(TjunctionD)
  T_conduction/1 -> Sum1/1, Mul5/1  "Transistor conduction losses (W)"
  Sum2/1 -> PEC_loss (W)/1  "Total inverter power switch losses (W)"
  Look-up-maps/3(Vd) -> Mux/8  "V_d0"
  UDC/1 -> "Modulation index "/2(UDC), Look-up-maps/2(Udc), Mux/3  "U_dc"
  Number of switches/1 -> Mul3/2, Mul5/2, Mul4/1, Mul2/2, Mul1/1
  Idle switch losses (W)/1 -> Mul3/1
  Mul3/1 -> Sum2/1
  Sum1/1 -> One Transistor losses/1
  Sum/1 -> One Diode losses/1
  Uphase_rms/1 -> "Modulation index "/1(Uphase_rms)  "U phase RMS"

== system EDR100_Model4/Transmission Vehicle-EM/Power flow/Energy Engine -> Wheel ==
  w_wheel : Inport
  T_wheel : Inport  Port=2
  gear_ratio : Inport  Port=3
  Constant1 : Constant  Value=P_GT0
  Constant2 : Constant  Value=inf
  Gain : Gain  Gain=e_GT  SaturateOnIntegerOverflow=on  OutDataTypeStr=Inherit: Same as input  ParamDataTypeStr=Inherit: Same as input
  Product2 : Product  Inputs=*/  InputSameDT=on  RndMeth=Zero  SaturateOnIntegerOverflow=on  OutDataTypeStr=Inherit: Same as first input
  Product3 : Product  Inputs=/*  InputSameDT=on  RndMeth=Zero  SaturateOnIntegerOverflow=on  OutDataTypeStr=Inherit: Same as first input
  Sum : Sum  InputSameDT=on  SaturateOnIntegerOverflow=on  OutDataTypeStr=Inherit: Same as first input
  Switch1 : Switch  Threshold=w_wheel_min
  T_trans+ : Outport  InitialOutput=0
  wires:
  gear_ratio/1 -> Gain/1
  Constant1/1 -> Product3/2
  Switch1/1 -> Product3/1
  Constant2/1 -> Switch1/3
  w_wheel/1 -> Switch1/1, Switch1/2
  Sum/1 -> Product2/1
  Product2/1 -> T_trans+/1
  Gain/1 -> Product2/2
  Product3/1 -> Sum/1
  T_wheel/1 -> Sum/2

== system EDR100_Model4/Transmission Vehicle-EM/Power flow/Energy Wheel -> Engine ==
  w_wheel : Inport
  T_wheel : Inport  Port=2
  gear_ratio : Inport  Port=3
  Constant1 : Constant  Value=P_GT0
  Constant2 : Constant  Value=inf
  Gain1 : Gain  Gain=e_GT  SaturateOnIntegerOverflow=on  OutDataTypeStr=Inherit: Same as input  ParamDataTypeStr=Inherit: Same as input
  Gain2 : Gain  Gain=1/e_GT  SaturateOnIntegerOverflow=on  OutDataTypeStr=Inherit: Same as input  ParamDataTypeStr=Inherit: Same as input
  Product2 : Product  Inputs=*/  InputSameDT=on  RndMeth=Zero  SaturateOnIntegerOverflow=on  OutDataTypeStr=Inherit: Same as first input
  Product3 : Product  Inputs=/*  InputSameDT=on  RndMeth=Zero  SaturateOnIntegerOverflow=on  OutDataTypeStr=Inherit: Same as first input
  Sum : Sum  InputSameDT=on  SaturateOnIntegerOverflow=on  OutDataTypeStr=Inherit: Same as first input
  Switch1 : Switch  Threshold=w_wheel_min
  T_trans- : Outport  InitialOutput=0
  wires:
  Gain1/1 -> Product3/1
  Sum/1 -> Product2/1
  Product3/1 -> Sum/2
  Product2/1 -> T_trans-/1
  Gain2/1 -> Product2/2
  T_wheel/1 -> Sum/1
  Constant1/1 -> Product3/2
  Switch1/1 -> Gain1/1
  Constant2/1 -> Switch1/3
  gear_ratio/1 -> Gain2/1
  w_wheel/1 -> Switch1/2, Switch1/1

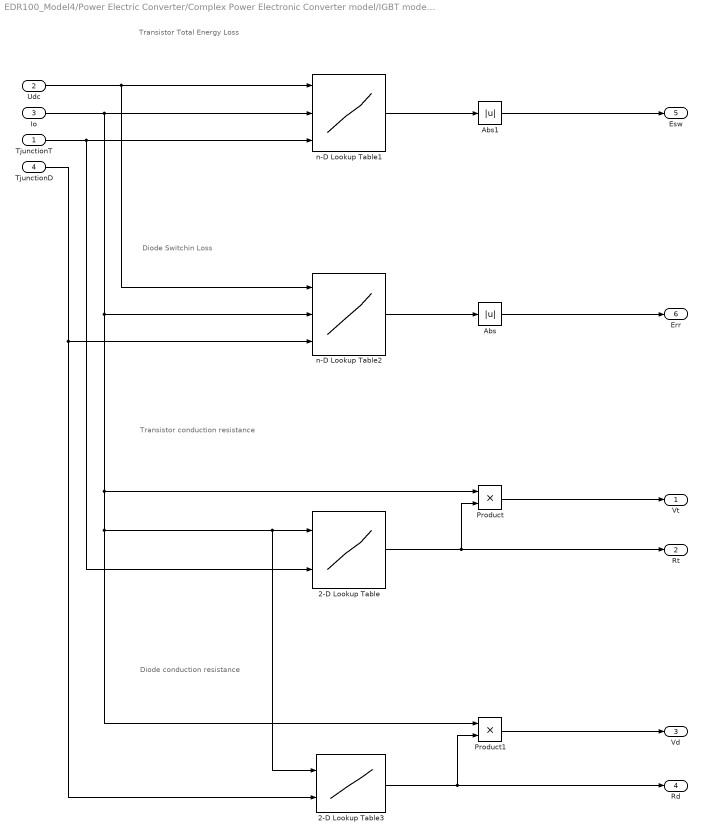
== system EDR100_Model4/Power Electric Converter/Complex Power Electronic Converter model/IGBT model/Look-up-maps ==
  note: Diode conduction resistance
  note: Transistor conduction resistance
  note: Transistor Total Energy Loss
  note: Diode Switchin Loss
  TjunctionT : Inport
  Udc : Inport  Port=2
  "Io " : Inport  Port=3
  TjunctionD : Inport  Port=4
  2-D Lookup Table : Lookup_n-D  BreakpointsForDimension1=PEC_i2  BreakpointsForDimension2=PEC_T2  Table=PEC_Rt_con  ExtrapMethod=Clip  InternalRulePriority=Speed  RndMeth=Simplest
      settings: InputPortMap=u0,u1
  2-D Lookup Table3 : Lookup_n-D  BreakpointsForDimension1=PEC_i2  BreakpointsForDimension2=PEC_T2  Table=PEC_Rd_con  ExtrapMethod=Clip  InternalRulePriority=Speed  RndMeth=Simplest
      settings: InputPortMap=u0,u1
  Abs : Abs  SaturateOnIntegerOverflow=off
  Abs1 : Abs  SaturateOnIntegerOverflow=off
  Product : Product
  Product1 : Product
  n-D Lookup Table1 : Lookup_n-D  NumberOfTableDimensions=3  BreakpointsForDimension1=PEC_v1  BreakpointsForDimension2=PEC_i1  BreakpointsForDimension3=PEC_T1  Table=PEC_J_ON_OFF_T  InternalRulePriority=Speed  RndMeth=Simplest
      settings: InputPortMap=u0,u1,u2
  n-D Lookup Table2 : Lookup_n-D  NumberOfTableDimensions=3  BreakpointsForDimension1=PEC_v1  BreakpointsForDimension2=PEC_i1  BreakpointsForDimension3=PEC_T1  Table=PEC_J_ON_OFF_D  ExtrapMethod=Clip  UseLastTableValue=on  InternalRulePriority=Speed  RndMeth=Simplest
      settings: InputPortMap=u0,u1,u2
  Vt : Outport  VectorParamsAs1DForOutWhenUnconnected=off
  Rt : Outport  Port=2  VectorParamsAs1DForOutWhenUnconnected=off
  Vd : Outport  Port=3  VectorParamsAs1DForOutWhenUnconnected=off
  Rd : Outport  Port=4  VectorParamsAs1DForOutWhenUnconnected=off
  Esw : Outport  Port=5  VectorParamsAs1DForOutWhenUnconnected=off
  Err : Outport  Port=6  VectorParamsAs1DForOutWhenUnconnected=off
  wires:
  2-D Lookup Table/1 -> Rt/1, Product/2
  TjunctionD/1 -> n-D Lookup Table2/3, 2-D Lookup Table3/2
  2-D Lookup Table3/1 -> Rd/1, Product1/2
  Product/1 -> Vt/1
  Udc/1 -> n-D Lookup Table1/1, n-D Lookup Table2/1
  TjunctionT/1 -> n-D Lookup Table1/3, 2-D Lookup Table/2
  "Io "/1 -> n-D Lookup Table1/2, n-D Lookup Table2/2, Product1/1, 2-D Lookup Table3/1, 2-D Lookup Table/1, Product/1
  n-D Lookup Table1/1 -> Abs1/1
  Product1/1 -> Vd/1
  n-D Lookup Table2/1 -> Abs/1
  Abs/1 -> Err/1
  Abs1/1 -> Esw/1

== system EDR100_Model4/Power Electric Converter/Complex Power Electronic Converter model/IGBT model/Modulation index  ==
  note: Definition of amplitude modulation index:
      | Range from [0 .. 1.15].
      | 1.0 means maximum modulation for tri-sine modulation.
      | 1.15 possible with PVM or THI.
  Uphase_rms : Inport
  UDC : Inport  Port=2
  Divide : Product  Inputs=*/
  Gain1 : Gain  Gain=2*sqrt(2)
  Mod : Outport
  wires:
  UDC/1 -> Divide/2
  Uphase_rms/1 -> Divide/1
  Divide/1 -> Gain1/1
  Gain1/1 -> Mod/1

== matlab function EDR100_Model4/Electric Machine/Overspeed and overtorque control/OverSpeed text ==
  data: u input
    function fcn(u)
    if u ~ 0
        %error('EM over-speed error!');
        fprintf(2, 'EM over-speed error! \n');
    end
end

== matlab function EDR100_Model4/Electric Machine/Overspeed and overtorque control/OverTorque text ==
  data: u input
function fcn(u)
    if u ~ 0
        %error('EM over-torque error! \n');
        fprintf(2, 'EM over-torque error! \n');
    end
end

== matlab function EDR100_Model4/Electrical Energy Storage System/Cell Electrical Model and Protection/Voltage protection ==
  data: Vhigh input; Vlow input; stop output; Vactual input
function stop = fcn(Vhigh,Vlow,Vactual)
    stop = 0;
    if Vactual > Vhigh
        fprintf(2, 'ESS cell over-voltage error!\n');
        stop = 1   
    end
    if Vactual < Vlow
        fprintf(2, 'ESS cell under-voltage error!\n');
        stop = 1   
    end
end

== matlab function EDR100_Model4/Electrical Energy Storage System/Cell Electrical Model and Protection/SOC protection ==
  data: SOC input; stop output
function stop = fcn(SOC)
    stop = 0;
    if SOC > 100
        fprintf(2, 'ESS over-charge error!\n');
        stop = 1   
    end
    if SOC < 0
        fprintf(2, 'ESS deep discharge error!\n');
        stop = 1   
    end
end

== matlab function EDR100_Model4/Electrical Energy Storage System/Cell Electrical Model and Protection/Peak current protection ==
  data: Imax input; Imin input; stop output; Iactual input
function stop = fcn(Imax,Imin,Iactual)
    stop = 0;
    if Iactual > Imax
        fprintf(2, 'ESS cell over-current discharge error!\n');
        stop = 1   
    end
    if Iactual < Imin
        fprintf(2, 'ESS cell over-current charge error!\n');
        stop = 1   
    end
end

== matlab function EDR100_Model4/Power Electric Converter/Phase over current protection ==
  data: Imax input; Irms input; stop output
function stop = fcn(Imax,Irms)
    stop = 0;
    if Irms > Imax
        fprintf(2, 'PEC over-current error!\n');
        stop = 1   
    end
end

== matlab function EDR100_Model4/Power Electric Converter/Phase over voltage protection ==
  data: V_max input; V_actual input; stop output
function stop = fcn(V_max,V_actual)
    stop = 0;
    if V_actual > V_max
        fprintf(2, 'PEC over-voltage error!\n');
        stop = 1   
    end
end
